simulink model "lqrmodel"  (R2023a)
settings: Solver=VariableStepAuto  StartTime=0.0  StopTime=10.0  RelTol=1e-3
undefined symbols (not defined in the file): A, B, C_l, C_m, g, I_noload, init, J_observer, K, K_int, K_m, K_x, l, m, min_sampling_time, potentiometer_linearity_percent, R_a, wave_amplitude, wave_period, x1_bar, x2_bar
settings Model: Creator=yunzh  LastModifiedBy=yunzh

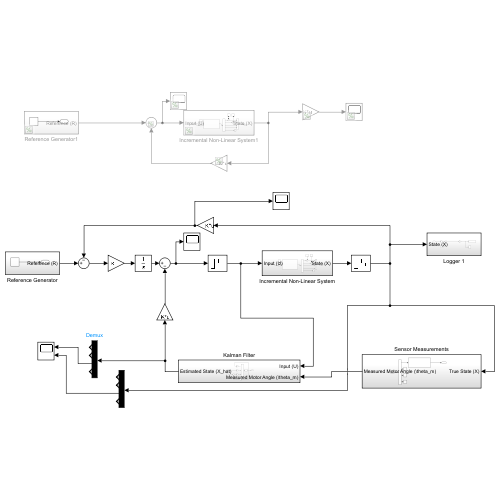
[thumbnail: Simulink's stored preview of the top-level diagram]
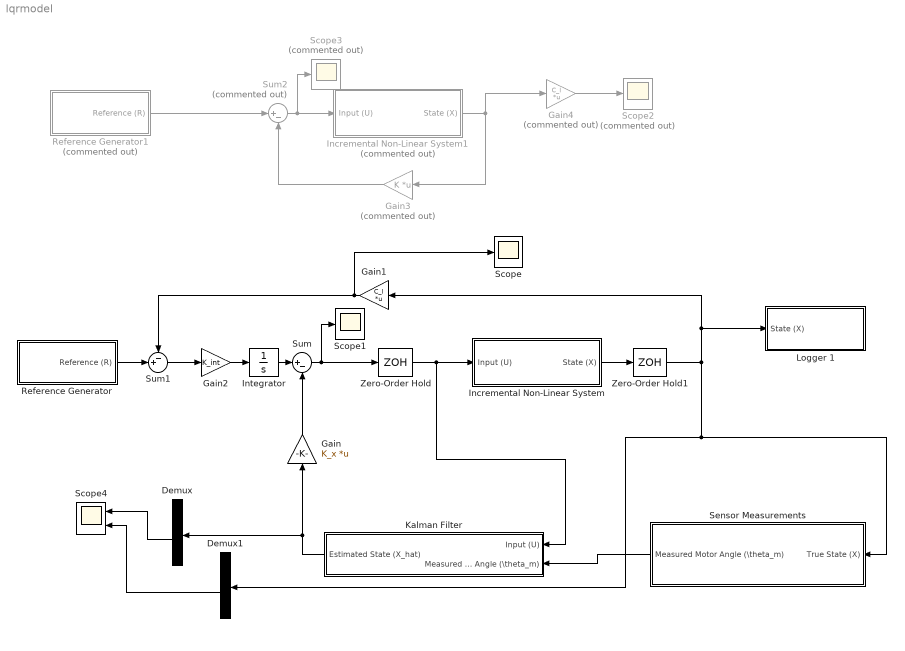
== system lqrmodel ==
  Demux : Demux
  Demux1 : Demux
  Gain : Gain  Gain=K_x  Multiplication=Matrix(K*u)
  Gain1 : Gain  Gain=C_l  Multiplication=Matrix(K*u)
  Gain2 : Gain  Gain=K_int
  Gain3 : Gain  Commented=on  Gain=K  Multiplication=Matrix(K*u)
  Gain4 : Gain  Commented=on  Gain=C_l  Multiplication=Matrix(K*u)
  Incremental Non-Linear System : Subsystem
  Incremental Non-Linear System1 : Subsystem  Commented=on
  Integrator : Integrator
  Kalman Filter : Subsystem
  Logger 1 : Subsystem
  Reference Generator : Subsystem
  Reference Generator1 : Subsystem  Commented=on
  Scope : Scope
  Scope1 : Scope
  Scope2 : Scope  Commented=on
  Scope3 : Scope  Commented=on
  Scope4 : Scope  NumInputPorts=2
  Sensor Measurements : Subsystem
  Sum : Sum  Inputs=|+-
  Sum1 : Sum  Inputs=-+|
  Sum2 : Sum  Commented=on  Inputs=|+-
  Zero-Order Hold : ZeroOrderHold  SampleTime=min_sampling_time
  Zero-Order Hold1 : ZeroOrderHold  SampleTime=min_sampling_time
  wires:
  Sum/1 -> Scope1/1, Zero-Order Hold/1
  Gain/1 -> Sum/2
  Incremental Non-Linear System/1(State (X)) -> Zero-Order Hold1/1
  Integrator/1 -> Sum/1
  Reference Generator/1(Reference (R)) -> Sum1/2
  Gain1/1 -> Scope/1, Sum1/1
  Sum1/1 -> Gain2/1
  Gain2/1 -> Integrator/1
  Incremental Non-Linear System1/1(State (X)) -> Gain4/1, Gain3/1
  Sum2/1 -> Scope3/1, Incremental Non-Linear System1/1(Input (U))
  Gain3/1 -> Sum2/2
  Gain4/1 -> Scope2/1
  Reference Generator1/1(Reference (R)) -> Sum2/1
  Zero-Order Hold/1 -> Kalman Filter/1(Input (U)), Incremental Non-Linear System/1(Input (U))
  Zero-Order Hold1/1 -> Demux1/1, Sensor Measurements/1(True State (X)), Logger 1/1(State (X)), Gain1/1
  Kalman Filter/1(Estimated State (X_hat)) -> Demux/1, Gain/1
  Sensor Measurements/1(Measured Motor Angle (\theta_m)) -> Kalman Filter/2(Measured Motor Angle (\theta_m))
  Demux/3 -> Scope4/1
  Demux1/3 -> Scope4/2

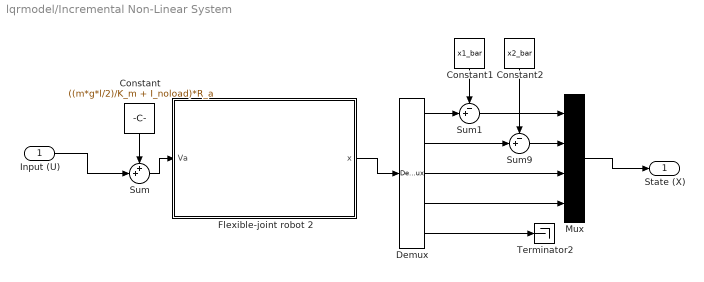
== system lqrmodel/Incremental Non-Linear System ==
  Input (U) : Inport
  Constant : Constant  Value=((m*g*l/2)/K_m + I_noload)*R_a
  Constant1 : Constant  Value=x1_bar
  Constant2 : Constant  Value=x2_bar
  Demux : Demux  Outputs=5
  Flexible-joint robot 2 : Subsystem
      mask Display: image('$imagefile'); % Use "Edit Image" on toolstrip to change.
  Mux : Mux
  Sum : Sum  Inputs=++|
  Sum1 : Sum  Inputs=-+|
  Sum9 : Sum  Inputs=-+|
  Terminator2 : Terminator
  State (X) : Outport
  wires:
  Flexible-joint robot 2/1(x) -> Demux/1
  Demux/1 -> Sum1/2
  Demux/2 -> Sum9/2
  Demux/5 -> Terminator2/1
  Sum/1 -> Flexible-joint robot 2/1(Va)
  Constant1/1 -> Sum1/1
  Sum9/1 -> Mux/2
  Constant2/1 -> Sum9/1
  Sum1/1 -> Mux/1
  Demux/4 -> Mux/4
  Demux/3 -> Mux/3
  Constant/1 -> Sum/1
  Input (U)/1 -> Sum/2
  Mux/1 -> State (X)/1

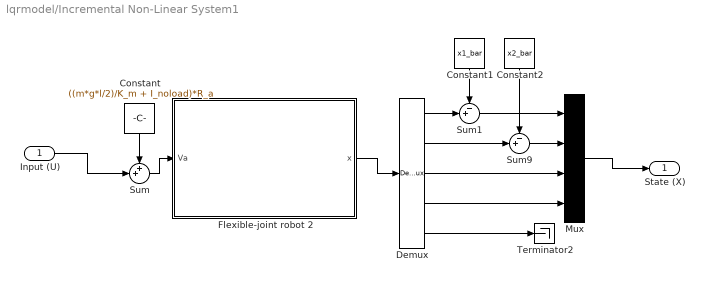
== system lqrmodel/Incremental Non-Linear System1 ==
  Input (U) : Inport
  Constant : Constant  Value=((m*g*l/2)/K_m + I_noload)*R_a
  Constant1 : Constant  Value=x1_bar
  Constant2 : Constant  Value=x2_bar
  Demux : Demux  Outputs=5
  Flexible-joint robot 2 : Subsystem
      mask Display: image('$imagefile'); % Use "Edit Image" on toolstrip to change.
  Mux : Mux
  Sum : Sum  Inputs=++|
  Sum1 : Sum  Inputs=-+|
  Sum9 : Sum  Inputs=-+|
  Terminator2 : Terminator
  State (X) : Outport
  wires:
  Flexible-joint robot 2/1(x) -> Demux/1
  Demux/1 -> Sum1/2
  Demux/2 -> Sum9/2
  Demux/5 -> Terminator2/1
  Sum/1 -> Flexible-joint robot 2/1(Va)
  Constant1/1 -> Sum1/1
  Sum9/1 -> Mux/2
  Constant2/1 -> Sum9/1
  Sum1/1 -> Mux/1
  Demux/4 -> Mux/4
  Demux/3 -> Mux/3
  Constant/1 -> Sum/1
  Input (U)/1 -> Sum/2
  Mux/1 -> State (X)/1

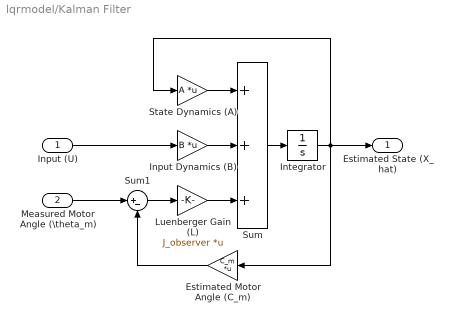
== system lqrmodel/Kalman Filter ==
  Input (U) : Inport
  Measured Motor Angle (\theta_m) : Inport  Port=2
  Estimated Motor Angle (C_m) : Gain  Gain=C_m  Multiplication=Matrix(K*u)
  Input Dynamics (B) : Gain  Gain=B  Multiplication=Matrix(K*u)
  Integrator : Integrator
  Luenberger Gain (L) : Gain  Gain=J_observer  Multiplication=Matrix(K*u)
  State Dynamics (A) : Gain  Gain=A  Multiplication=Matrix(K*u)
  Sum : Sum  Inputs=+++
  Sum1 : Sum  Inputs=|+-
  Estimated State (X_hat) : Outport
  wires:
  Input (U)/1 -> Input Dynamics (B)/1
  Input Dynamics (B)/1 -> Sum/2
  Luenberger Gain (L)/1 -> Sum/3
  Estimated Motor Angle (C_m)/1 -> Sum1/2
  Sum/1 -> Integrator/1
  Sum1/1 -> Luenberger Gain (L)/1
  Integrator/1 -> Estimated State (X_hat)/1, State Dynamics (A)/1, Estimated Motor Angle (C_m)/1
  State Dynamics (A)/1 -> Sum/1
  Measured Motor Angle (\theta_m)/1 -> Sum1/1

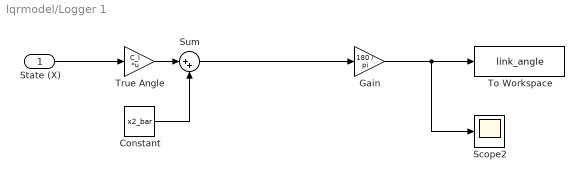
== system lqrmodel/Logger 1 ==
  State (X) : Inport
  Constant : Constant  Value=x2_bar
  Gain : Gain  Gain=180 / pi
  Scope2 : Scope
  Sum : Sum  Inputs=|++
  To Workspace : ToWorkspace  VariableName=link_angle  SaveFormat=Timeseries  SampleTime=-1
  True Angle : Gain  Gain=C_l  Multiplication=Matrix(K*u)
  wires:
  State (X)/1 -> True Angle/1
  True Angle/1 -> Sum/1
  Sum/1 -> Gain/1
  Gain/1 -> Scope2/1, To Workspace/1
  Constant/1 -> Sum/2

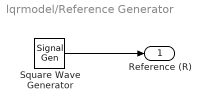
== system lqrmodel/Reference Generator ==
  Square Wave Generator : SignalGenerator  WaveForm=square  Amplitude=wave_amplitude  Frequency=1 / wave_period
  Reference (R) : Outport
  wires:
  Square Wave Generator/1 -> Reference (R)/1

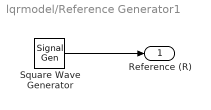
== system lqrmodel/Reference Generator1 ==
  Square Wave Generator : SignalGenerator  WaveForm=square  Amplitude=wave_amplitude  Frequency=1 / wave_period
  Reference (R) : Outport
  wires:
  Square Wave Generator/1 -> Reference (R)/1

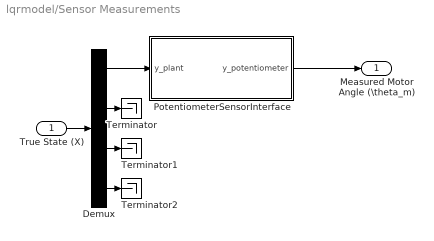
== system lqrmodel/Sensor Measurements ==
  True State (X) : Inport
  Demux : Demux
  PotentiometerSensorInterface : Subsystem  TreatAsAtomicUnit=on
      mask Display: image('$imagefile'); % Use "Edit Image" on toolstrip to change.
  Terminator : Terminator
  Terminator1 : Terminator
  Terminator2 : Terminator
  Measured Motor Angle (\theta_m) : Outport
  wires:
  Demux/1 -> PotentiometerSensorInterface/1(y_plant)
  True State (X)/1 -> Demux/1
  Demux/2 -> Terminator/1
  Demux/3 -> Terminator1/1
  Demux/4 -> Terminator2/1
  PotentiometerSensorInterface/1(y_potentiometer) -> Measured Motor Angle (\theta_m)/1

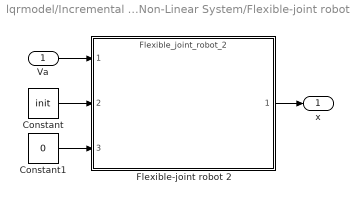
== system lqrmodel/Incremental Non-Linear System/Flexible-joint robot 2 ==
  Va : Inport
  Constant : Constant  Value=init
  Constant1 : Constant  Value=0
  Flexible-joint robot 2 : ModelReference  ModelNameDialog=Flexible_joint_robot_2  ModelReferenceVersion=1.65  CopyOfModelProtected=on
  x : Outport
  wires:
  Va/1 -> Flexible-joint robot 2/1
  Constant1/1 -> Flexible-joint robot 2/3
  Constant/1 -> Flexible-joint robot 2/2
  Flexible-joint robot 2/1 -> x/1

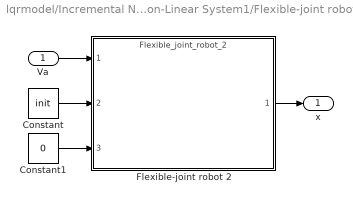
== system lqrmodel/Incremental Non-Linear System1/Flexible-joint robot 2 ==
  Va : Inport
  Constant : Constant  Value=init
  Constant1 : Constant  Value=0
  Flexible-joint robot 2 : ModelReference  ModelNameDialog=Flexible_joint_robot_2  ModelReferenceVersion=1.65  CopyOfModelProtected=on
  x : Outport
  wires:
  Va/1 -> Flexible-joint robot 2/1
  Constant1/1 -> Flexible-joint robot 2/3
  Constant/1 -> Flexible-joint robot 2/2
  Flexible-joint robot 2/1 -> x/1

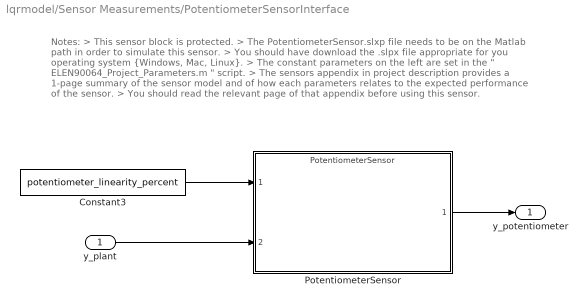
== system lqrmodel/Sensor Measurements/PotentiometerSensorInterface ==
  note: Notes:
      | > This sensor block is protected.
      | > The PotentiometerSensor.slxp file needs to be on the Matlab path in order to simulate this sensor.
      | > You should have download the .slpx file appropriate for you operating system {Windows, Mac, Linux}.
      | > The constant parameters on the left are set in the " ELEN90064_Project_Parameters.m " script.
      | > The sensors appendix in project description provides a 1-page summary of the sensor model and of how each parameters relates to the expected performance of the sensor.
      | > You should read the relevant page of that appendix before using this sensor.
  y_plant : Inport
  Constant3 : Constant  Value=potentiometer_linearity_percent
  PotentiometerSensor : ModelReference  ModelNameDialog=PotentiometerSensor.slxp  ModelReferenceVersion=1.21  CopyOfModelProtected=on
  y_potentiometer : Outport
  wires:
  y_plant/1 -> PotentiometerSensor/2
  Constant3/1 -> PotentiometerSensor/1
  PotentiometerSensor/1 -> y_potentiometer/1
